simulink model "WEankle_controllerMaarten_TimingPerturb"  (R2021b)
settings: Solver=FixedStepDiscrete  StartTime=0.0  StopTime=inf  FixedStep=sampleTime  RelTol=1e-3
undefined symbols (not defined in the file or in its folder): DiscIntNeverNeededParam, forceplate
libraries: simulink x17, WE2_library x8, dspsigops x6, dspfdesign x3
(part 3 of 3)

== matlab function WEankle_controllerMaarten_TimingPerturb/GetAnkleAngleStanding/MATLAB Function ==
  data: q input; qLeft output; start input; caltime_s input; qRight output
function [qLeft, qRight] = EncoderOffset_GeyerModel(q, start, caltime_s)
% q = joint angle
% start = boolean indicate start callibration is triggered
% caltime_s = total callibration time

qLeft = f_EncoderOffset_GeyerModel(q(1),start,caltime_s);
qRight = f_EncoderOffset_GeyerModel(q(2),start,caltime_s);

== matlab function WEankle_controllerMaarten_TimingPerturb/Ankle Controller/MATLAB Function5 ==
  data: e0 input; G input; SolGains output; COMd input
function SolGains  = CombineSoleusGains(e0,G,COMd)
% input arguments:

SolGains = [e0; G; COMd];

== matlab function WEankle_controllerMaarten_TimingPerturb/ForcePlate/Calibration/MATLAB Function ==
  data: left input; left_calib output; right input; start input; right_calib output; caltime_s input
function [left_calib, right_calib] = calibrateOffset(left, right, start, caltime_s)
persistent calibrated
persistent offcum_left
persistent offcum_right
persistent counter
persistent nosamp

if(isempty(calibrated))
   calibrated = false;
   offcum_left = left*0;
   offcum_right = right*0;
   counter = 0;
   nosamp = max(1, floor(caltime_s*1000));
end

if(start == 1)
    counter = 0;
    calibrated = false;
    offcum_left = left*0;
    offcum_right = right*0;
    nosamp = max(1, floor(caltime_s*1000));
end

if(calibrated)
    left_calib = left - offcum_left;
    right_calib = right - offcum_right;
else
    if(~calibrated)
        counter = counter + 1;
        offcum_left = offcum_left + left/(nosamp);
        offcum_right = offcum_right + right/(nosamp);
        if(counter >= nosamp)
            calibrated = true;
        end
    end
    left_calib = left;
    right_calib = right;
end

== matlab function WEankle_controllerMaarten_TimingPerturb/Ankle Controller/Eventdetection/COP detection (treadmill)/MATLAB Function2 ==
  data: x input; y output; OmegaFilter input; sampleTime input
function y = Filter2ndOrder(x, OmegaFilter, sampleTime)
%#codegen

persistent yd_prev y_prev;
if isempty(yd_prev)
    yd_prev = zeros(6,1); 
    y_prev = zeros(6,1);  %Derivative of the above signal
end

% Do 2nd order filtering with given omega and zeta=0.7; input of filter
% is vel_inc_sampleTime_unfilt; output is y (we assign to vel_inc_s
% later). 
if OmegaFilter==0 || isinf(OmegaFilter)
    y = x;
    y_prev = y;
    yd_prev = zeros(6,1); 
else
    zeta = 0.7;
    ydd = OmegaFilter^2 * (x - y_prev) - 2*zeta*OmegaFilter* yd_prev;
    yd = yd_prev + ydd * sampleTime;
    y = y_prev + yd * sampleTime;

    y_prev = y; yd_prev = yd;
end

== matlab function WEankle_controllerMaarten_TimingPerturb/Ankle Controller/COMverror and perturbation/TriggerPerturbation/Perturbation sync gait phase1/TimeBetweenPert ==
  data: TimeBetweenPert input; timesvector input; Allow output; Delivered input
function Allow = fcn(TimeBetweenPert,timesvector,Delivered)
% To randomize the time between perturbations (min 6s)
persistent i 
persistent TimeSelector 
persistent flagfirst %flag to indicate first time
if isempty(i)
    i = 1;
    flagfirst = 1;
end
if Delivered == 1 && ~flagfirst %Perturbation delivered. Go to next element of timesVector avoiding a false entrance the first time
    i = i+1;
end
%% Assign new time
len = length(timesvector);
if i > len %reset the index when all perturbations from the vector are done
    i = 1;
end
TimeSelector = timesvector(i);

if TimeSelector < 6
    TimeSelector = 6;
end
%% Allow new perturbation or not
if TimeBetweenPert >= TimeSelector
    Allow = 1;
else
    Allow = 0;
end
%%
flagfirst = 0;

== matlab function WEankle_controllerMaarten_TimingPerturb/Ankle Controller/Eventdetection/Subsystem/MATLAB Function ==
  data: f input; y output; nf input; nf_1 input; th input
function y = fcn(f,nf,nf_1,th)

maxCounter = 200; %time to wait in zero
persistent counter
persistent out
if isempty(counter)
    counter = maxCounter+1;
    out = f;
end

if (nf == 0) && (nf_1 < -50)
    out = 0;
    counter = 0;
else
    counter = counter+1;
    if counter > maxCounter
        if (f > -th) && (f < th) && (nf == 0)
            out = 0;
        else
            out = f;
        end
    end
end

y = out;

== matlab function WEankle_controllerMaarten_TimingPerturb/Ankle Controller/Eventdetection/StrideTimeEstimator/MATLAB Function3 ==
  data: fLeftCross input; fLeftThresh input; phase_left output; fRightCross input; fRightThresh input; time input; phase_right output; SingleL input; SingleR input; reset input
function [phase_left, phase_right] = fcn(fLeftCross, fLeftThresh, fRightCross, fRightThresh, time, SingleL, SingleR, reset)

persistent time_heel2heel_right
persistent time_heellast_right
persistent tdm_right
persistent time_heel2heel_left
persistent time_heellast_left
persistent tdm_left
persistent  phase_left2
persistent  phase_right2

if(isempty(time_heel2heel_left) || reset==1)
   time_heel2heel_right = zeros(4,1);
   time_heellast_right = -1e5;
   tdm_right = 0.1;
   
   time_heel2heel_left = zeros(4,1);
   time_heellast_left = -1e5;
   tdm_left = 0.1;
   
    phase_left2 = 0; %Used to reset the left phase when prepositioning of left leg is detected (SingleL 1 to 0)
    phase_right2 = 0; %Used to reset the right phase when prepositioning of right leg is detected (SingleR 1 to 0)
end
%% left
phase_left = (time - time_heellast_left)/(tdm_left+eps)*100 - phase_left2;
% if(fLeftCross~=0||(phase_left>100&&fLeftThresh==1))

if(SingleR)
    phase_left2 = phase_left;
end
if((fLeftCross~=0||(phase_left>100&&fLeftThresh==1)))
    td_new  = time - time_heellast_left;
    phase_left2 = 0;
    if((td_new>0.8*tdm_left)||any(time_heel2heel_left>10))
        time_heellast_left = time;
        time_heel2heel_left(2:end) = time_heel2heel_left(1:end-1);
        time_heel2heel_left(1) = td_new;
        tdm_left = mean(time_heel2heel_left);
    end
end


%% right
phase_right = (time - time_heellast_right)/(tdm_right+eps)*100 - phase_right2;
% if(fRightCross~=0||(phase_right>100&&fRightThresh==1))
if(SingleL)
    phase_right2 = phase_right;
end
if(fRightCross~=0||(phase_right>100&&fRightThresh==1))
    td_new  = time - time_heellast_right;
    phase_right2 = 0;
    if((td_new>0.8*tdm_right)||any(time_heel2heel_right>10))
        time_heellast_right = time;
        time_heel2heel_right(2:end) = time_heel2heel_right(1:end-1);
        time_heel2heel_right(1) = td_new;
        tdm_right = mean(time_heel2heel_right);
    end
end
